simulink model "Ejer1P2"  (R2024b)
settings: Solver=VariableStepAuto  StartTime=0.0  StopTime=10.0  RelTol=1e-3
settings Model: Creator=lopez  LastModifiedBy=lopez

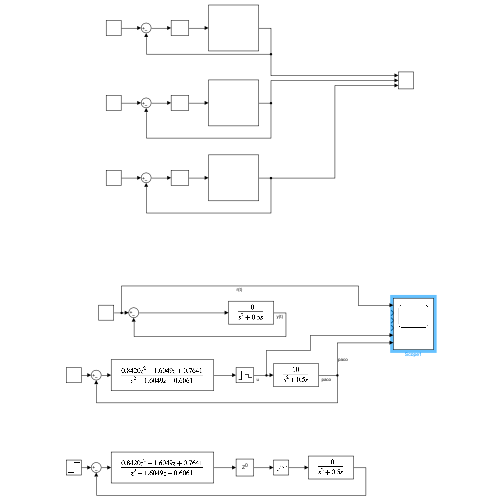
[thumbnail: Simulink's stored preview of the top-level diagram]
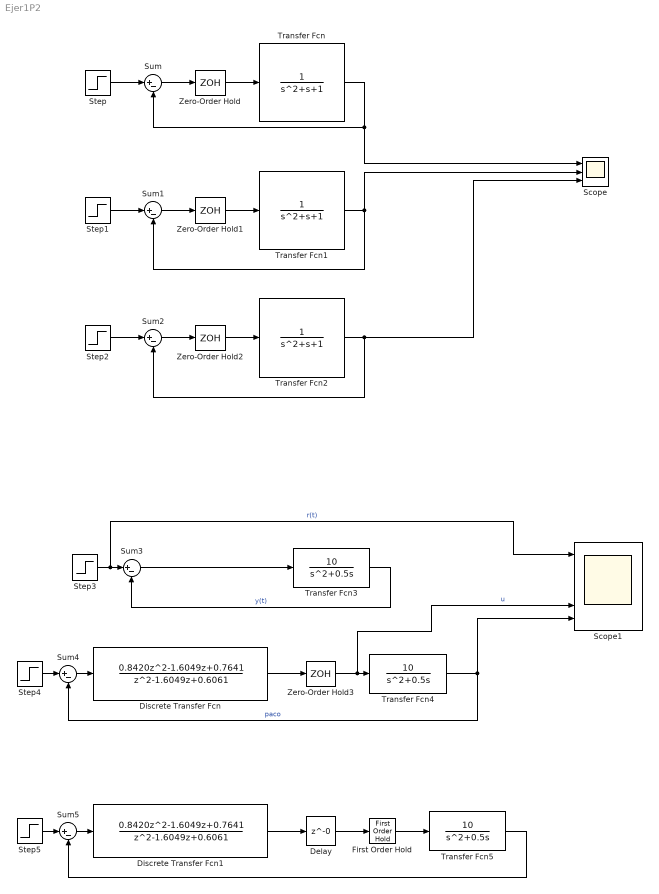
== system Ejer1P2 ==
  Delay : Delay  DelayLength=0  SampleTime=0.1
  Discrete Transfer Fcn : DiscreteTransferFcn  Numerator="[0.8420  -1.6049  0.7641]"  Denominator=[1 -1.6049 0.6061]
  Discrete Transfer Fcn1 : DiscreteTransferFcn  Numerator=[0.8420 -1.6049 0.7641]  Denominator=[1 -1.6049 0.6061]
  First Order Hold : FirstOrderHold  ErrorTolerance=inf
  Scope : Scope  NumInputPorts=3
  Scope1 : Scope  NumInputPorts=6
  Step : Step  SampleTime=0
  Step1 : Step  SampleTime=0
  Step2 : Step  SampleTime=0
  Step3 : Step  Time=0  Before=1  SampleTime=0
  Step4 : Step  Time=0  Before=1  SampleTime=0
  Step5 : Step  Time=0  Before=1  SampleTime=0
  Sum{,1..5} (6 alike) : Sum  Inputs=|+-
  Transfer Fcn : TransferFcn  Denominator=[1 1 1]
  Transfer Fcn1 : TransferFcn  Denominator=[1 1 1]
  Transfer Fcn2 : TransferFcn  Denominator=[1 1 1]
  Transfer Fcn3 : TransferFcn  Numerator=[10]  Denominator=[1 0.5 0]
  Transfer Fcn4 : TransferFcn  Numerator=[10]  Denominator=[1 0.5 0]
  Transfer Fcn5 : TransferFcn  Numerator=[10]  Denominator=[1 0.5 0]
  Zero-Order Hold : ZeroOrderHold  SampleTime=0.01
  Zero-Order Hold1 : ZeroOrderHold  SampleTime=0.1
  Zero-Order Hold2 : ZeroOrderHold
  Zero-Order Hold3 : ZeroOrderHold  SampleTime=-1
  wires:
  Step/1 -> Sum/1
  Sum/1 -> Zero-Order Hold/1
  Zero-Order Hold/1 -> Transfer Fcn/1
  Sum1/1 -> Zero-Order Hold1/1
  Zero-Order Hold1/1 -> Transfer Fcn1/1
  Step1/1 -> Sum1/1
  Sum2/1 -> Zero-Order Hold2/1
  Zero-Order Hold2/1 -> Transfer Fcn2/1
  Step2/1 -> Sum2/1
  Transfer Fcn1/1 -> Scope/2, Sum1/2
  Transfer Fcn2/1 -> Sum2/2, Scope/3
  Transfer Fcn/1 -> Sum/2, Scope/1
  Sum3/1 -> Transfer Fcn3/1
  Transfer Fcn3/1 -> Sum3/2  "y(t)"
  Step3/1 -> Scope1/1, Sum3/1  "r(t)"
  Discrete Transfer Fcn/1 -> Zero-Order Hold3/1
  Zero-Order Hold3/1 -> Scope1/5, Transfer Fcn4/1  "u"
  Transfer Fcn4/1 -> Scope1/6, Sum4/2  "paco"
  Sum4/1 -> Discrete Transfer Fcn/1
  Step4/1 -> Sum4/1
  Sum5/1 -> Discrete Transfer Fcn1/1
  Step5/1 -> Sum5/1
  First Order Hold/1 -> Transfer Fcn5/1
  Delay/1 -> First Order Hold/1
  Discrete Transfer Fcn1/1 -> Delay/1
  Transfer Fcn5/1 -> Sum5/2
